simulink model "dcmotor"  (Simulink 6.0)
settings: Solver=ode45  StartTime=0.0  StopTime=10.0  RelTol=1e-3
values from neighbouring files (symbols this model uses):
  b = 0.5    [dcmotor.m]
  J = 2    [dcmotor.m]
  ka = 54    [dcmotor.m]
  kb = 0.1    [dcmotor.m]
  km = 10    [dcmotor.m]
  kt = 1    [dcmotor.m]
  La = 0.5    [dcmotor.m]
  Ra = 1    [dcmotor.m]
settings Model: LastModifiedBy=Administrator

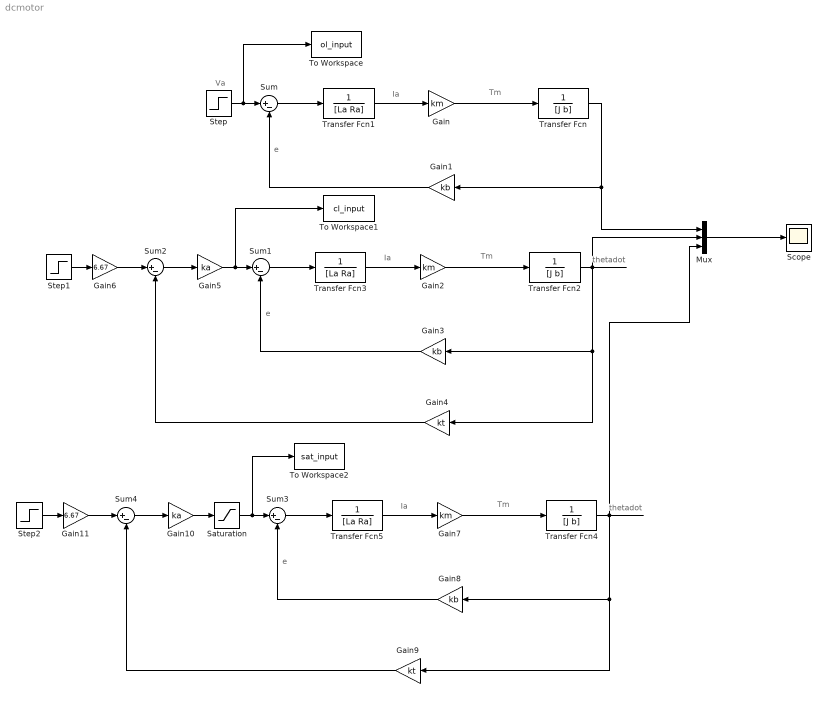
== system dcmotor ==
  note: Va
  note: e
  note: Ia
  note: Tm
  note: e
  note: Ia
  note: Tm
  note: thetadot
  note: e
  note: Ia
  note: Tm
  note: thetadot
  Gain : Gain  Gain=km
  Gain1 : Gain  Orientation=left  Gain=kb
  Gain10 : Gain  Gain=ka
  Gain11 : Gain  Gain=6.67
  Gain2 : Gain  Gain=km
  Gain3 : Gain  Orientation=left  Gain=kb
  Gain4 : Gain  Orientation=left  Gain=kt
  Gain5 : Gain  Gain=ka
  Gain6 : Gain  Gain=6.67
  Gain7 : Gain  Gain=km
  Gain8 : Gain  Orientation=left  Gain=kb
  Gain9 : Gain  Orientation=left  Gain=kt
  Mux : Mux  Inputs=3
  Saturation : Saturate  UpperLimit=10  LowerLimit=-10
  Scope : Scope
  Step : Step  SampleTime=0
  Step1 : Step  SampleTime=0
  Step2 : Step  SampleTime=0
  Sum{,1..4} (5 alike) : Sum  Inputs=|+-
  To Workspace : ToWorkspace  VariableName=ol_input  SampleTime=-1  SaveFormat=Array
  To Workspace1 : ToWorkspace  VariableName=cl_input  SampleTime=-1  SaveFormat=Array
  To Workspace2 : ToWorkspace  VariableName=sat_input  SampleTime=-1  SaveFormat=Array
  Transfer Fcn : TransferFcn  Denominator=[J b]
  Transfer Fcn1 : TransferFcn  Denominator=[La Ra]
  Transfer Fcn2 : TransferFcn  Denominator=[J b]
  Transfer Fcn3 : TransferFcn  Denominator=[La Ra]
  Transfer Fcn4 : TransferFcn  Denominator=[J b]
  Transfer Fcn5 : TransferFcn  Denominator=[La Ra]
  wires:
  Transfer Fcn1/1 -> Gain/1
  Gain/1 -> Transfer Fcn/1
  Transfer Fcn/1 -> Gain1/1, Mux/1
  Gain1/1 -> Sum/2
  Sum/1 -> Transfer Fcn1/1
  Step/1 -> Sum/1, To Workspace/1
  Transfer Fcn3/1 -> Gain2/1
  Gain2/1 -> Transfer Fcn2/1
  Transfer Fcn2/1 -> Gain3/1, Gain4/1, Mux/2
  Gain3/1 -> Sum1/2
  Sum1/1 -> Transfer Fcn3/1
  Gain5/1 -> Sum1/1, To Workspace1/1
  Sum2/1 -> Gain5/1
  Gain4/1 -> Sum2/2
  Mux/1 -> Scope/1
  Step1/1 -> Gain6/1
  Gain6/1 -> Sum2/1
  Transfer Fcn5/1 -> Gain7/1
  Gain7/1 -> Transfer Fcn4/1
  Transfer Fcn4/1 -> Gain8/1, Gain9/1, Mux/3
  Gain8/1 -> Sum3/2
  Sum3/1 -> Transfer Fcn5/1
  Gain10/1 -> Saturation/1
  Sum4/1 -> Gain10/1
  Gain9/1 -> Sum4/2
  Step2/1 -> Gain11/1
  Gain11/1 -> Sum4/1
  Saturation/1 -> Sum3/1, To Workspace2/1
